simulink model "x2_lidar_core"  (R2022b)
settings: Solver=FixedStepAuto  StartTime=0.0  StopTime=inf  FixedStep=0.01  RelTol=1e-3
InitFcn:
  | Ts = 0.01;
libraries: instrumentseriallib x2
settings Model: Creator=System-10  LastModifiedBy=System-10
settings ModelReferenceCC: PropagateVarSize=Only when enabling

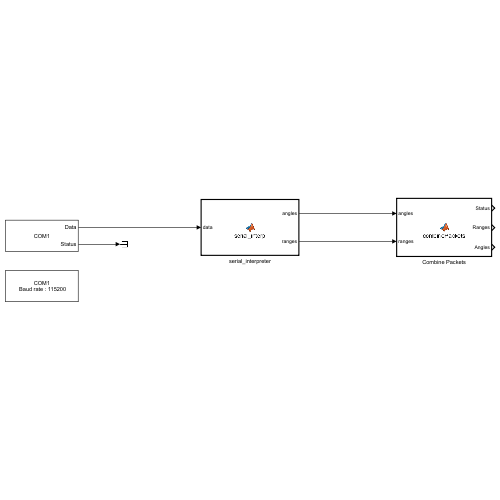
[thumbnail: Simulink's stored preview of the top-level diagram]
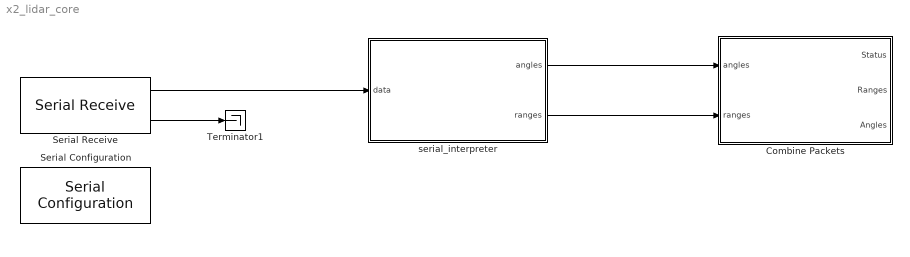
== system x2_lidar_core ==
  Combine Packets : MATLAB Function  TreatAsAtomicUnit=on
  Serial Configuration : instrumentseriallib/Serial Configuration  Priority=-200000  PortSel=COM1  Port=COM1  ComPort=COM1  BaudRate=115200  DataBits=8  Parity=none  StopBits=1  ByteOrder=little-endian  FlowControl=none  Timeout=10  SimulateUsing=Interpreted execution  BlockInModel=on  aMode=1
  Serial Receive : instrumentseriallib/Serial Receive  Priority=1  PortSel=COM1  Port=COM1  ComPort=COM1  DataType=uint8  SaveDataType=uint8  ToggleHeader=off  Header=[170 85]  ToggleTerminator=off  Terminator=<none>  CustomTerminator=[]  InputFormat=Column major  ToggleDataSize=on  DataSize=[1 2000]  EnableBlockingMode=off  ActionDataUnavailable=Output last received value  ActionWhenDataUnavailable=Output last received value  CustomValue=111  SampleTime=Ts  SimulateUsing=Interpreted execution  BlockInModel=on  aMode=1
  Terminator1 : Terminator
  serial_interpreter : MATLAB Function  TreatAsAtomicUnit=on
  wires:
  Serial Receive/1 -> serial_interpreter/1(data)
  Serial Receive/2 -> Terminator1/1
  serial_interpreter/2(ranges) -> Combine Packets/2(ranges)
  serial_interpreter/1(angles) -> Combine Packets/1(angles)

== matlab function x2_lidar_core/Combine Packets ==
  settings: updateMethod=DISCRETE  sampleTime=Ts
  data: Status output boolean; Ranges output size=[1 400]; angles input; Angles output size=[1 400]; ranges input
function [Status,Ranges,Angles]  = combinePackets(angles,ranges)
    persistent count; 
    persistent elemAngles;
    persistent elemRanges;
    
    if sum(angles) == 0
        Angles = zeros(1,400);
        Ranges = zeros(1,400);
        Status = boolean(0);
        return;
    end

    if isempty(count)
        count = 0;
        elemAngles = zeros(1,400);
        elemRanges = zeros(1,400);
    end
        
    for i = 1:length(angles)
        elemAngles(i+count) = angles(i);
        elemRanges(i+count) = ranges(i);
    end
    if count < (length(elemAngles)-length(angles))
        count = count + length(angles);
        Angles = zeros(1,400);
        Ranges = zeros(1,400);
        Status = boolean(0);
    else
        count = 0;
        %Current Angles as 1x400 array [rad].
        Angles = deg2rad(elemAngles);
        %Current Ranges as 1x400 array [meter].
        Ranges = elemRanges;
        Status = boolean(1);
    end
end

== matlab function x2_lidar_core/serial_interpreter ==
  settings: updateMethod=DISCRETE  sampleTime=Ts
  data: data input; angles output; ranges output
function [angles,ranges] = serial_interp(data)

    persistent lastData;
    persistent indices;
    persistent currentIdx;
    persistent Si;
    persistent AngleSi;

    if isempty(lastData)
        lastData = uint8(zeros(1,size(data,2)));
        Si = zeros(1, 40);
        AngleSi = zeros(1, 40);
    end
    if isempty(indices) || ~isequal(data, lastData)
        indices = find(data==170 | data==85);
        indices = indices(diff(indices) == 1);
        indices = indices(diff(indices) == 90);
        currentIdx = 1;
        lastData = data;
    end

    if currentIdx <= numel(indices)
         FSA = double(bitshift ...
             (double ...
             (bitor ...
             (bitshift ...
             (uint16(data(1, indices(currentIdx)+5)), 8), uint16(data(1, indices(currentIdx)+4) ...
             ), ...
             'uint16')), ...
             -1) / 64);
         LSA = double(bitshift ...
             (double ...
             (bitor ...
             (bitshift ...
             (uint16(data(1, indices(currentIdx)+7)), 8), uint16(data(1, indices(currentIdx)+6) ...
             ), ...
             'uint16')), ...
             -1) / 64);
         
         diffAngle = mod((LSA - FSA),360);

         for j = 1:80
             if mod(j, 2) == 0
                Si(j / 2) = double(bitor ...
                    (bitshift ...
                    (uint16(data(1, (indices(currentIdx)+9)+j)), 8), ...
                    uint16(data(1, (indices(currentIdx)+9)+j-1)), 'uint16') ...
                    );
                if Si(j / 2) == 0
                    AngleSi(j / 2) = ((diffAngle / (40 - 1)) * ((j / 2) - 1) + FSA);
                else
                    AngleSi(j / 2) = ((diffAngle / (40 - 1)) * ((j / 2) - 1) + FSA) + atan(21.8*((155.3-Si((j / 2)))/(155.3*Si((j / 2)))));
                end
             end
         end
        %Current Angles as 1x40 array [deg].
        angles = AngleSi;
    
        %Current Ranges as 1x40 array [meter].
        ranges = Si / 4000;
        currentIdx = currentIdx + 1;
    else
        angles = zeros(1, 40);
        ranges = zeros(1, 40);
    end
end
